simulink model "acciones_control"  (R2020b)
settings: Solver=VariableStepAuto  StartTime=0.0  StopTime=50  RelTol=1e-3
libraries: simulink x1
settings Model: Creator=Acer  LastModifiedBy=Acer

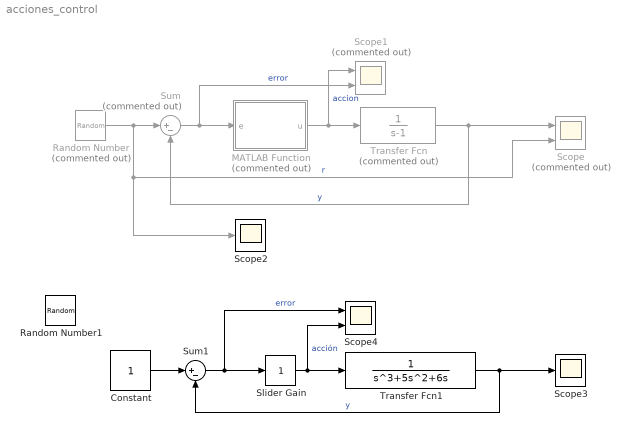
== system acciones_control ==
  Constant : Constant  VectorParams1D=off  SampleTime=-1
  MATLAB Function : MATLAB Function  Commented=on  TreatAsAtomicUnit=on
  Random Number : RandomNumber  Commented=on  SampleTime=7
  Random Number1 : RandomNumber  SampleTime=20
  Scope : Scope  Commented=on  NumInputPorts=2
  Scope1 : Scope  Commented=on  NumInputPorts=2
  Scope2 : Scope
  Scope3 : Scope
  Scope4 : Scope  NumInputPorts=2
  Slider Gain : simulink/Math Operations/Slider Gain  gain=1  low=0  high=100
  Sum : Sum  Commented=on  Inputs=|+-
  Sum1 : Sum  Inputs=|+-
  Transfer Fcn : TransferFcn  Commented=on  Denominator=[1 -1]
  Transfer Fcn1 : TransferFcn  Denominator=[1 5 6 0]
  wires:
  Transfer Fcn/1 -> Scope/1, Sum/2  "y"
  Sum/1 -> Scope1/2, MATLAB Function/1(e)  "error"
  MATLAB Function/1(u) -> Scope1/1, Transfer Fcn/1  "accion"
  Random Number/1 -> Scope/2, Scope2/1, Sum/1  "r"
  Slider Gain/1 -> Scope4/2, Transfer Fcn1/1  "acción"
  Sum1/1 -> Scope4/1, Slider Gain/1  "error"
  Transfer Fcn1/1 -> Scope3/1, Sum1/2  "y"
  Constant/1 -> Sum1/1

== matlab function acciones_control/MATLAB Function ==
  data: e input; u output
function u = cont_on_off(e)
if e>=0
    u=1;
else
    u=0;
end
